simulink model "BINAY_ESPIRITU_BLOCKDIAGRAMREDUCTION"  (R2023b)
settings: Solver=VariableStepAuto  StartTime=0.0  StopTime=1  RelTol=1e-3
settings Model: Creator=ninabinay  LastModifiedBy=ninabinay
settings DebuggingCC: AlgebraicLoopMsg=none

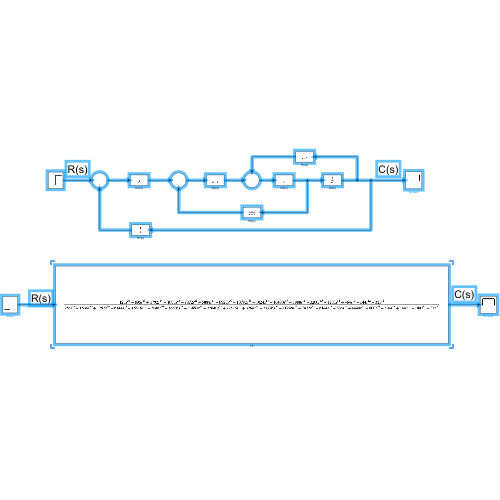
[thumbnail: Simulink's stored preview of the top-level diagram]
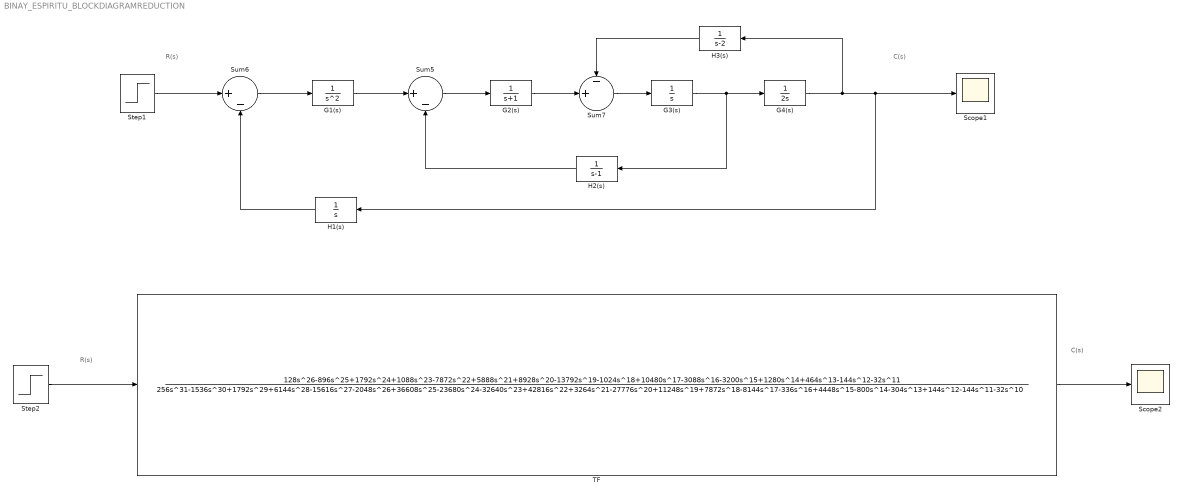
== system BINAY_ESPIRITU_BLOCKDIAGRAMREDUCTION ==
  note: R(s)
  note: C(s)
  note: R(s)
  note: C(s)
  G1(s) : TransferFcn  Denominator=[1 0 0]
  G2(s) : TransferFcn  Denominator=[1 1]
  G3(s) : TransferFcn  Denominator=[1 0]
  G4(s) : TransferFcn  Denominator=[2 0]
  H1(s) : TransferFcn  Denominator=[1 0]
  H2(s) : TransferFcn  Denominator=[1 -1]
  H3(s) : TransferFcn  Denominator=[1 -2]
  Scope1 : Scope
  Scope2 : Scope
  Step1 : Step  Time=0  SampleTime=0
  Step2 : Step  Time=0  SampleTime=0
  Sum5 : Sum  Inputs=|+-
  Sum6 : Sum  Inputs=|+-
  Sum7 : Sum  Inputs=-+|
  TF : TransferFcn  Numerator=[128 -896 1792 1088 -7872 5888 8928 -13792 -1024 10480 -3088 -3200 1280 464 -144 -32 0 0 0 0 0 0 0 0 0 0 0]  Denominator=[256 -1536 1792 6144 -15616 -2048 36608 -23680 -32640 42816 3264 -27776 11248 7872 -8144 -336 4448 -800 -304 144 -144 -32 0 0 0 0 0 0 0 0 0 0]
  wires:
  Step1/1 -> Sum6/1
  Sum6/1 -> G1(s)/1
  G1(s)/1 -> Sum5/1
  Sum5/1 -> G2(s)/1
  G2(s)/1 -> Sum7/2
  Sum7/1 -> G3(s)/1
  G3(s)/1 -> H2(s)/1, G4(s)/1
  G4(s)/1 -> H3(s)/1, H1(s)/1, Scope1/1
  H3(s)/1 -> Sum7/1
  H2(s)/1 -> Sum5/2
  H1(s)/1 -> Sum6/2
  TF/1 -> Scope2/1
  Step2/1 -> TF/1
